simulink model "keyEventModifier"  (R2016b)
settings: Solver=VariableStepAuto  StartTime=0.0  StopTime=10.0  RelTol=1e-3
settings Model: DataDictionary=DataDictionary.sldd  Creator=Taeke  LastModifiedBy=Taeke

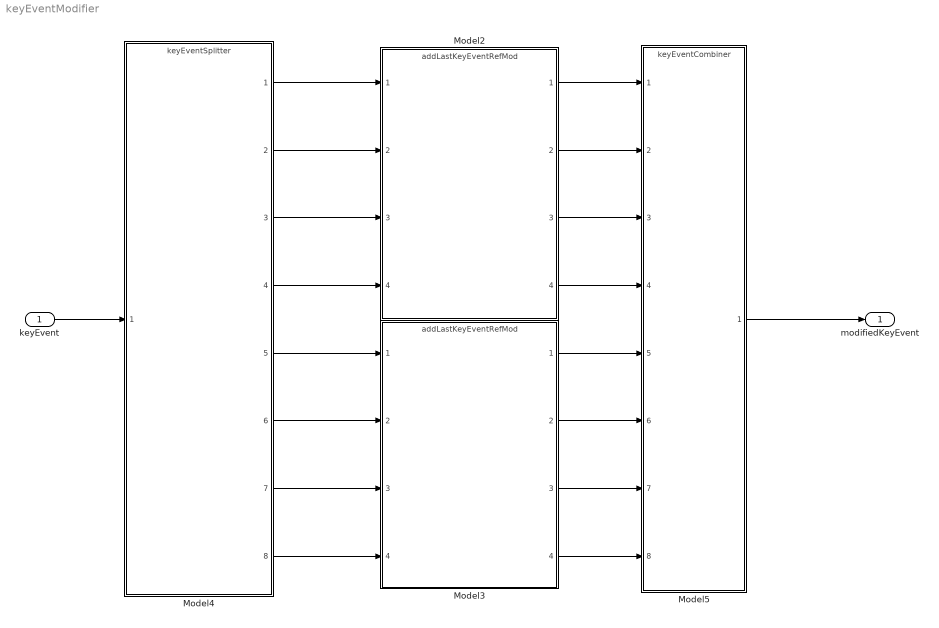
== system keyEventModifier ==
  keyEvent : Inport  OutDataTypeStr=Bus: keyEventTotal  BusOutputAsStruct=on
  Model2 : ModelReference  ModelNameDialog=addLastKeyEventRefMod.slx  SimulationMode=Normal  ModelReferenceVersion=1.23
  Model3 : ModelReference  ModelNameDialog=addLastKeyEventRefMod.slx  SimulationMode=Normal  ModelReferenceVersion=1.23
  Model4 : ModelReference  ModelNameDialog=keyEventSplitter.slx  SimulationMode=Normal  ModelReferenceVersion=1.3
  Model5 : ModelReference  ModelNameDialog=keyEventCombiner.slx  SimulationMode=Normal  ModelReferenceVersion=1.6
  modifiedKeyEvent : Outport  OutDataTypeStr=Bus: keyEventTotal
  wires:
  Model3/1 -> Model5/5
  Model3/2 -> Model5/6
  Model4/7 -> Model3/3
  Model4/6 -> Model3/2
  Model4/4 -> Model2/4
  Model4/3 -> Model2/3
  Model4/2 -> Model2/2
  Model5/1 -> modifiedKeyEvent/1
  Model4/8 -> Model3/4
  Model4/1 -> Model2/1
  Model4/5 -> Model3/1
  keyEvent/1 -> Model4/1
  Model3/3 -> Model5/7
  Model3/4 -> Model5/8
  Model2/4 -> Model5/4
  Model2/3 -> Model5/3
  Model2/2 -> Model5/2
  Model2/1 -> Model5/1
